simulink model "ex3p2"  (R2016b)
settings: Solver=VariableStepAuto  StartTime=0.0  StopTime=0.4  RelTol=1e-3
InitFcn:
  | alpha=30;
libraries: powerlib x12, powerlib_meascontrol x5, simulink x4
settings Model: Creator=user  LastModifiedBy=user

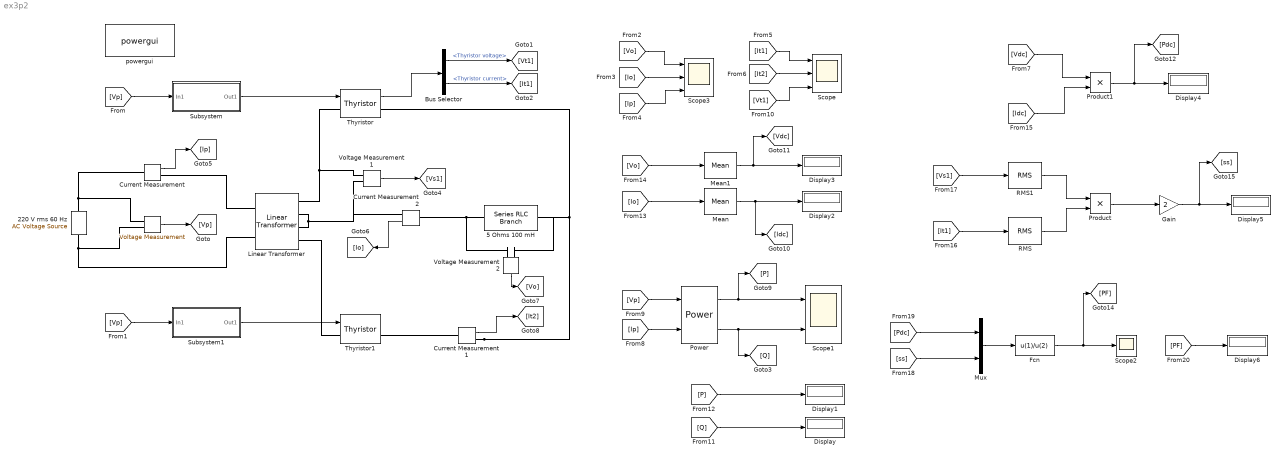
== system ex3p2 ==
  " " : powerlib/Measurements/Voltage Measurement  PhasorSimulation=off  OutputType=Complex  PSBequivalent=0
  220 V rms 60 Hz : powerlib/Electrical Sources/AC Voltage Source  Amplitude=220*sqrt(2)  Phase=0  Frequency=60  SampleTime=0  Measurements=None  BusType=swing  Pref=10e3  Qref=0  Qmin=-inf  Qmax=+inf
  5 Ohms 100 mH : powerlib/Elements/Series RLC Branch  LConnTagsString=__new0  RConnTagsString=__new0  BranchType=RL  Resistance=5  Inductance=100e-3  SetiL0=off  InitialCurrent=0  Capacitance=1e-6  Setx0=off  InitialVoltage=0  Measurements=None
  Bus Selector : BusSelector  OutputSignals=Thyristor voltage,Thyristor current
  Current Measurement : powerlib/Measurements/Current Measurement  PhasorSimulation=off  OutputType=Complex  PSBequivalent=0
  Current Measurement1 : powerlib/Measurements/Current Measurement  PhasorSimulation=off  OutputType=Complex  PSBequivalent=0
  Current Measurement2 : powerlib/Measurements/Current Measurement  PhasorSimulation=off  OutputType=Complex  PSBequivalent=0
  Display{,1..6} (7 alike) : Display
  Fcn : Fcn  Expr=u(1)/u(2)
  Gain : Gain  Gain=2
  Linear Transformer : powerlib/Elements/Linear Transformer  UNITS=pu  NominalPower=[ 100e3 60 ]  winding1="[220  0.002  0.08 ]"  winding2="[266.5  0.002  0.08 ]"  ThreeWindings=on  winding3=[266.5 0.002 0.08 ]  RmLm=[ 500 500 ]  Measurements=None  DataType=off
  Mean : powerlib_meascontrol/Measurements/Mean  Freq=60  Vinit=0  Ts=0
  Mean1 : powerlib_meascontrol/Measurements/Mean  Freq=60  Vinit=0  Ts=0
  Mux : Mux  Inputs=2
  Power : powerlib_meascontrol/Measurements/Power  Freq=60  Vinit=[1, 0]  Iinit=[1, 0]  Ts=0
  Product : Product
  Product1 : Product
  RMS : powerlib_meascontrol/Measurements/RMS  TrueRMS=on  Freq=60  RMSInit=120  Ts=0
  RMS1 : powerlib_meascontrol/Measurements/RMS  TrueRMS=on  Freq=60  RMSInit=120  Ts=0
  Scope : Scope  NumInputPorts=3
  Scope1 : Scope  NumInputPorts=2
  Scope2 : Scope
  Scope3 : Scope  NumInputPorts=3
  Subsystem : Subsystem
  Subsystem1 : Subsystem
  Thyristor : powerlib/Power Electronics/Thyristor  Ron=0.001  Lon=0  Vf=0.8  IC=0  Rs=500  Cs=250e-9  Measurements=on
  Thyristor1 : powerlib/Power Electronics/Thyristor  Ron=0.001  Lon=0  Vf=0.8  IC=0  Rs=500  Cs=250e-9  Measurements=on
  Voltage Measurement1 : powerlib/Measurements/Voltage Measurement  PhasorSimulation=off  OutputType=Complex  PSBequivalent=0
  Voltage Measurement2 : powerlib/Measurements/Voltage Measurement  PhasorSimulation=off  OutputType=Complex  PSBequivalent=0
  powergui : powerlib/powergui  Priority=1  SimulationMode=Continuous  SolverType=Tustin/Backward Euler (TBE)  SampleTime=50e-6  frequency=60  SPID=off  DisableSnubberDevices=off  DisableRonSwitches=off  DisableVfSwitches=off  SwTol=0  DisplayEquations=off  Interpol=off  ExternalGateDelay=off  methode=off  Ts=10  FunctionMessages=off  echomessages=off  HookPort=off  EnableUseOfTLC=off  x0status=blocks  frequencyindice=60  Pbase=100e6  ErrMax=1e-4  Iterations=50  UnitsV=kV  UnitsW=MW  buscounter=0  RestoreLinks=warning  ResistiveCurrentMeasurement=off  Frange=[0:2:500]  Ylog=off  Xlog=on  ShowGrid=off  save=off  variable=ZData  structure=0  ZoomFFT=off  StartTime=0.0  cycles=1  DisplayStyle=1  fundamental=60  FreqAxis=off  MaxFrequency=1000  frequencyindicesteady=1  RmsSteady=1  display=off
  wires:
  Subsystem/1(Out1) -> Thyristor/1
  Subsystem1/1(Out1) -> Thyristor1/1
  " "/1 -> [Vp]
  [Vp] -> Subsystem1/1(In1)
  [Vp] -> Subsystem/1(In1)
  Thyristor/1 -> Bus Selector/1
  Bus Selector/1 -> [Vt1]  "<Thyristor voltage>"
  Bus Selector/2 -> [It1]  "<Thyristor current>"
  Voltage Measurement1/1 -> [Vs1]
  Current Measurement1/1 -> [It2]
  Voltage Measurement2/1 -> [Vo]
  Current Measurement2/1 -> [Io]
  Current Measurement/1 -> [Ip]
  [Vo] -> Scope3/1
  [Io] -> Scope3/2
  [Ip] -> Scope3/3
  [It1] -> Scope/1
  [It2] -> Scope/2
  [Vt1] -> Scope/3
  [Vp] -> Power/1
  [Ip] -> Power/2
  Power/1 -> [P], Scope1/1
  Power/2 -> [Q], Scope1/2
  Mean1/1 -> [Vdc], Display3/1
  Mean/1 -> [Idc], Display2/1
  [Vo] -> Mean1/1
  [Io] -> Mean/1
  [P] -> Display1/1
  [Q] -> Display/1
  [Vs1] -> RMS1/1
  [It1] -> RMS/1
  RMS1/1 -> Product/1
  RMS/1 -> Product/2
  Product/1 -> Gain/1
  Gain/1 -> [ss], Display5/1
  [Idc] -> Product1/2
  [Vdc] -> Product1/1
  Product1/1 -> [Pdc], Display4/1
  [Pdc] -> Mux/1
  [ss] -> Mux/2
  [PF] -> Display6/1
  Mux/1 -> Fcn/1
  Fcn/1 -> [PF], Scope2/1
  connections:
  220 V rms 60 Hz/RConn1 -- " "/LConn1 -- Current Measurement/LConn1
  220 V rms 60 Hz/LConn1 -- " "/LConn2 -- Linear Transformer/LConn2
  Linear Transformer/RConn3 -- Voltage Measurement1/LConn2 -- Current Measurement2/RConn1 -- Linear Transformer/RConn2
  Linear Transformer/RConn1 -- Voltage Measurement1/LConn1 -- Thyristor/LConn1
  5 Ohms 100 mH/LConn1 -- Voltage Measurement2/LConn2 -- Current Measurement2/LConn1
  Current Measurement1/RConn1 -- 5 Ohms 100 mH/RConn1 -- Voltage Measurement2/LConn1 -- Thyristor/RConn1
  Current Measurement/RConn1 -- Linear Transformer/LConn1
  Linear Transformer/RConn4 -- Thyristor1/LConn1
  Current Measurement1/LConn1 -- Thyristor1/RConn1

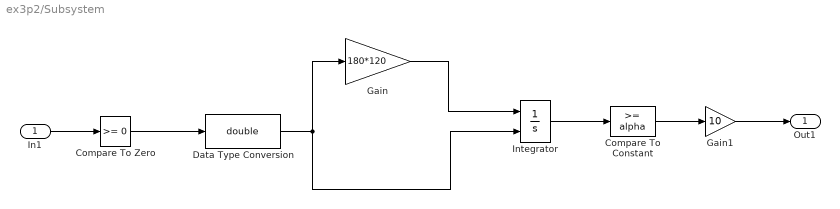
== system ex3p2/Subsystem ==
  In1 : Inport
  Compare To Constant : simulink/Logic and Bit Operations/Compare To Constant  relop=>=  const=alpha  OutDataTypeStr=boolean
  Compare To Zero : simulink/Logic and Bit Operations/Compare To Zero  relop=>=  OutDataTypeStr=boolean
  Data Type Conversion : DataTypeConversion  OutDataTypeStr=double
  Gain : Gain  Gain=180*120
  Gain1 : Gain  Gain=10
  Integrator : Integrator  ExternalReset=falling
  Out1 : Outport
  wires:
  In1/1 -> Compare To Zero/1
  Compare To Zero/1 -> Data Type Conversion/1
  Gain/1 -> Integrator/1
  Data Type Conversion/1 -> Gain/1, Integrator/2
  Integrator/1 -> Compare To Constant/1
  Compare To Constant/1 -> Gain1/1
  Gain1/1 -> Out1/1

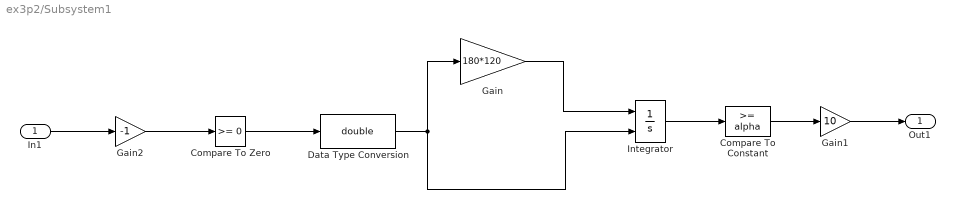
== system ex3p2/Subsystem1 ==
  In1 : Inport
  Compare To Constant : simulink/Logic and Bit Operations/Compare To Constant  relop=>=  const=alpha  OutDataTypeStr=boolean
  Compare To Zero : simulink/Logic and Bit Operations/Compare To Zero  relop=>=  OutDataTypeStr=boolean
  Data Type Conversion : DataTypeConversion  OutDataTypeStr=double
  Gain : Gain  Gain=180*120
  Gain1 : Gain  Gain=10
  Gain2 : Gain  Gain=-1
  Integrator : Integrator  ExternalReset=falling
  Out1 : Outport
  wires:
  Compare To Zero/1 -> Data Type Conversion/1
  Gain/1 -> Integrator/1
  Data Type Conversion/1 -> Gain/1, Integrator/2
  Integrator/1 -> Compare To Constant/1
  Compare To Constant/1 -> Gain1/1
  Gain1/1 -> Out1/1
  In1/1 -> Gain2/1
  Gain2/1 -> Compare To Zero/1
